simulink model "TVModel"  (R2022a)
settings: Solver=FixedStepDiscrete  StartTime=0.0  StopTime=10.0  FixedStep=0.02  MaxStep=0.01  RelTol=1e-3
undefined symbols (not defined in the file or in its folder): MB, TV, TV_OLD
libraries: simulink x22, simulink_extras x14, slpidlib x8, fuzblock x5, controlLib x4, dspstat3 x4, eeGeneralControl x3, cstblocks x3, eeSlidingModeController x1, sharedTrackingLibrary x1
(part 3 of 8)

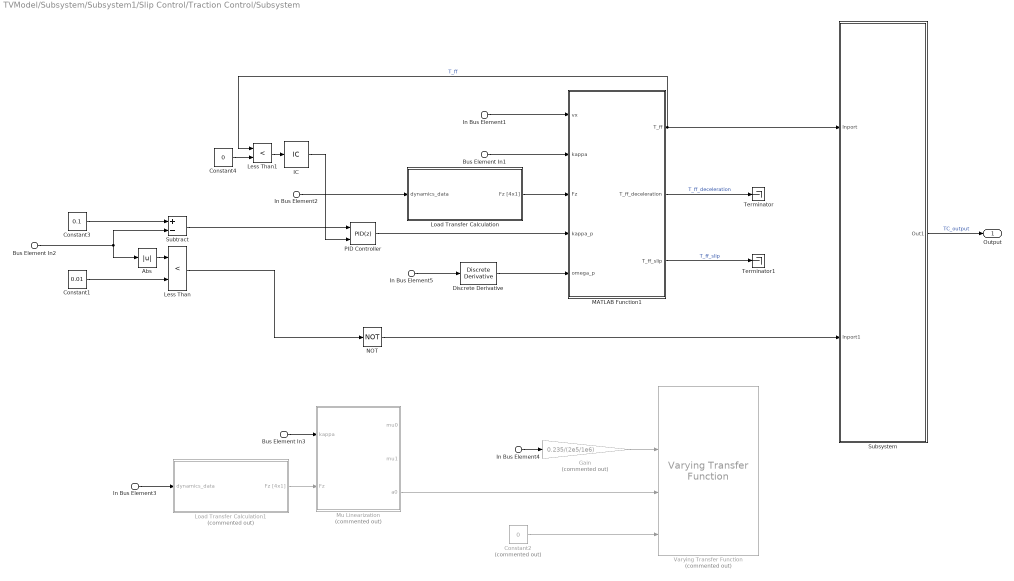
== system TVModel/Subsystem/Subsystem1/Slip Control/Traction Control/Subsystem ==
  In Bus Element2 : Inport  PortName=dynamics_data
  In Bus Element3 : Inport  PortName=dynamics_data
  In Bus Element1 : Inport  PortName=dynamics_data  Element=vx
  In Bus Element4 : Inport  PortName=dynamics_data  Element=vx
  In Bus Element5 : Inport  PortName=dynamics_data  Element=omega_wheels
  Bus Element In1 : Inport  Port=2  PortName=slip_ratio
  Bus Element In2 : Inport  Port=2  PortName=slip_ratio
  Bus Element In3 : Inport  Port=2  PortName=slip_ratio
  Abs : Abs  SaturateOnIntegerOverflow=off
  Constant1 : Constant  Value=0.01
  Constant2 : Constant  Commented=on  Value=0
  Constant3 : Constant  Value=0.1
  Constant4 : Constant  Value=0
  Discrete Derivative : simulink/Discrete/Discrete Derivative  gainval=1.0  ICPrevScaledInput=0.0  OutMin=[]  OutMax=[]  OutDataType=fixdt(1, 16)  OutScaling=2^-10  DoSatur=off
  Gain : Gain  Commented=on  Gain=0.235/(2e5/1e6)
  IC : InitialCondition
  Less Than : RelationalOperator  Operator=<  OutDataTypeStr=boolean  RndMeth=Simplest  InputSameDT=off
  Less Than1 : RelationalOperator  Operator=<  OutDataTypeStr=boolean  RndMeth=Simplest  InputSameDT=off
  Load Transfer Calculation : Subsystem
  Load Transfer Calculation1 : Subsystem  Commented=on
  MATLAB Function1 : MATLAB Function  TreatAsAtomicUnit=on
  Mu Linearization : MATLAB Function  Commented=on  TreatAsAtomicUnit=on
  NOT : Logic  Operator=NOT  IconShape=distinctive  AllPortsSameDT=off  OutDataTypeStr=boolean
  PID Controller : slpidlib/PID Controller  Controller=PID  Form=Parallel  TimeDomain=Discrete-time  UseExternalTs=off  SampleTime=-1  IntegratorMethod=Forward Euler  FilterMethod=Forward Euler  ControllerParametersSource=internal  P=1/(0.02*3)  I=100  UseKiTs=off  D=0  N=100  UseFilter=on  TunerSelectOption=Transfer Function Based (PID Tuner App)  InitialConditionSource=internal  InitialConditionForIntegrator=0  InitialConditionForFilter=0  DifferentiatorICPrevScaledInput=0  ExternalReset=level  TrackingMode=off  Kt=1  LimitOutput=on  SatLimitsSource=internal  UpperSaturationLimit=+20  LowerSaturationLimit=-20  LinearizeAsGain=on  AntiWindupMode=clamping  Kb=1  POutMin=[]  POutMax=[]  IOutMin=[]  IOutMax=[]  DOutMin=[]  DOutMax=[]  NOutMin=[]  NOutMax=[]  SumOutMin=[]  SumOutMax=[]  SaturationOutMin=[]  SaturationOutMax=[]  PParamMin=[]  PParamMax=[]  IParamMin=[]  IParamMax=[]  DParamMin=[]  DParamMax=[]  NParamMin=[]  NParamMax=[]  KbParamMin=[]  KbParamMax=[]  KtParamMin=[]  KtParamMax=[]  KbOutMin=[]  KbOutMax=[]  KtOutMin=[]  KtOutMax=[]  IntegratorOutMin=[]  IntegratorOutMax=[]  FilterOutMin=[]  FilterOutMax=[]  SumI1OutMin=[]  SumI1OutMax=[]  SumI2OutMin=[]  SumI2OutMax=[]  SumI3OutMin=[]  SumI3OutMax=[]  SumI4OutMin=[]  SumI4OutMax=[]  SumDOutMin=[]  SumDOutMax=[]  DifferentiatorOutMin=[]  DifferentiatorOutMax=[]  FilterDiffOutCoefMin=[]  FilterDiffOutCoefMax=[]  ReciprocalOutMin=[]  ReciprocalOutMax=[]  SumDenOutMin=[]  SumDenOutMax=[]  SumNumOutMin=[]  SumNumOutMax=[]  DivideOutMin=[]  DivideOutMax=[]  UdiffTsProdOutMin=[]  UdiffTsProdOutMax=[]  NTsProdOutMin=[]  NTsProdOutMax=[]  UintegralTsProdOutMin=[]  UintegralTsProdOutMax=[]  UngainTsProdOutMin=[]  UngainTsProdOutMax=[]  IntegratorContinuousStateAttributes=''  IntegratorStateMustResolveToSignalObject=off  IntegratorRTWStateStorageClass=Auto  FilterContinuousStateAttributes=''  FilterStateMustResolveToSignalObject=off  FilterRTWStateStorageClass=Auto  ParallelPVariant=InternalParameters  IdealPVariant=Disabled  IVariant=InternalParameters  DVariant=InternalParameters  IntegratorVariant=Discrete  SatVariant=Enabled  AWVariant=DiscClampingParallel  PCopyVariant=Disabled  TRVariant=Disabled  FdbkBlocksVariant=Forward  IdealPFdbkVariant=Disabled  SatFdbkVariant=Disabled  DerivativeFilterVariant=ForwardEulerFilter  NVariant=InternalParameters  NCopyVariant=Disabled  FilterICVariant=InternalICsFilter  IntegratorICVariant=InternalICs  ExternalResetVariant=ExternalReset  TRSumVariant=Passthrough  SumFdbkVariant=Disabled  SumVariant=Sum_PID  TsampFilterVariant=InternalTs  TsampNgainVariant=Passthrough  TsampIntegralVariant=Passthrough  ExternalSaturationOutDataTypeStr=Inherit: Same as second input  aMode=0
  Subsystem : Subsystem
  Subtract : Sum  Inputs=+-
  Terminator : Terminator
  Terminator1 : Terminator
  Varying Transfer Function : cstblocks/Linear Parameter Varying/Varying Transfer Function  Commented=on  N=1
  Output : Outport
  wires:
  Load Transfer Calculation/1(Fz [4x1]) -> MATLAB Function1/3(Fz)
  MATLAB Function1/1(T_ff) -> Less Than1/1, Subsystem/1(Inport)  "T_ff"
  Bus Element In1/1 -> MATLAB Function1/2(kappa)
  In Bus Element1/1 -> MATLAB Function1/1(vx)
  In Bus Element2/1 -> Load Transfer Calculation/1(dynamics_data)
  Bus Element In2/1 -> Subtract/2, Abs/1
  Constant3/1 -> Subtract/1
  Abs/1 -> Less Than/1
  Constant1/1 -> Less Than/2
  Subtract/1 -> PID Controller/1
  Bus Element In3/1 -> Mu Linearization/1(kappa)
  Load Transfer Calculation1/1(Fz [4x1]) -> Mu Linearization/2(Fz)
  In Bus Element3/1 -> Load Transfer Calculation1/1(dynamics_data)
  Constant2/1 -> Varying Transfer Function/4
  In Bus Element4/1 -> Gain/1
  Gain/1 -> Varying Transfer Function/2
  Mu Linearization/3(a0) -> Varying Transfer Function/3
  In Bus Element5/1 -> Discrete Derivative/1
  MATLAB Function1/2(T_ff_deceleration) -> Terminator/1  "T_ff_deceleration"
  MATLAB Function1/3(T_ff_slip) -> Terminator1/1  "T_ff_slip"
  Discrete Derivative/1 -> MATLAB Function1/5(omega_p)
  PID Controller/1 -> MATLAB Function1/4(kappa_p)
  NOT/1 -> Subsystem/2(Inport1)
  Subsystem/1(Out1) -> Output/1  "TC_output"
  Constant4/1 -> Less Than1/2
  Less Than1/1 -> IC/1
  Less Than/1 -> NOT/1
  IC/1 -> PID Controller/2

== system TVModel/Subsystem/Subsystem1/Slip Control/Traction Control/Subsystem1 ==
  In Bus Element2 : Inport  PortName=dynamics_data
  In Bus Element3 : Inport  PortName=dynamics_data
  In Bus Element1 : Inport  PortName=dynamics_data  Element=vx
  In Bus Element4 : Inport  PortName=dynamics_data  Element=vx
  In Bus Element5 : Inport  PortName=dynamics_data  Element=omega_wheels
  Bus Element In1 : Inport  Port=2  PortName=slip_ratio
  Bus Element In2 : Inport  Port=2  PortName=slip_ratio
  Bus Element In3 : Inport  Port=2  PortName=slip_ratio
  Abs : Abs  SaturateOnIntegerOverflow=off
  Constant1 : Constant  Value=0.01
  Constant2 : Constant  Commented=on  Value=0
  Constant3 : Constant  Value=-0.1
  Discrete Derivative : simulink/Discrete/Discrete Derivative  gainval=1.0  ICPrevScaledInput=0.0  OutMin=[]  OutMax=[]  OutDataType=fixdt(1, 16)  OutScaling=2^-10  DoSatur=off
  Gain : Gain  Commented=on  Gain=0.235/(2e5/1e6)
  Less Than : RelationalOperator  Operator=<  OutDataTypeStr=boolean  RndMeth=Simplest  InputSameDT=off
  Load Transfer Calculation : Subsystem
  Load Transfer Calculation1 : Subsystem  Commented=on
  MATLAB Function1 : MATLAB Function  TreatAsAtomicUnit=on
  Mu Linearization : MATLAB Function  Commented=on  TreatAsAtomicUnit=on
  NOT : Logic  Operator=NOT  IconShape=distinctive  AllPortsSameDT=off  OutDataTypeStr=boolean
  PID Controller : slpidlib/PID Controller  Controller=PID  Form=Parallel  TimeDomain=Discrete-time  UseExternalTs=off  SampleTime=-1  IntegratorMethod=Forward Euler  FilterMethod=Forward Euler  ControllerParametersSource=internal  P=1/(0.02*3)  I=100  UseKiTs=off  D=0  N=100  UseFilter=on  TunerSelectOption=Transfer Function Based (PID Tuner App)  InitialConditionSource=internal  InitialConditionForIntegrator=0  InitialConditionForFilter=0  DifferentiatorICPrevScaledInput=0  ExternalReset=level  TrackingMode=off  Kt=1  LimitOutput=on  SatLimitsSource=internal  UpperSaturationLimit=-5  LowerSaturationLimit=-20  LinearizeAsGain=on  AntiWindupMode=clamping  Kb=1  POutMin=[]  POutMax=[]  IOutMin=[]  IOutMax=[]  DOutMin=[]  DOutMax=[]  NOutMin=[]  NOutMax=[]  SumOutMin=[]  SumOutMax=[]  SaturationOutMin=[]  SaturationOutMax=[]  PParamMin=[]  PParamMax=[]  IParamMin=[]  IParamMax=[]  DParamMin=[]  DParamMax=[]  NParamMin=[]  NParamMax=[]  KbParamMin=[]  KbParamMax=[]  KtParamMin=[]  KtParamMax=[]  KbOutMin=[]  KbOutMax=[]  KtOutMin=[]  KtOutMax=[]  IntegratorOutMin=[]  IntegratorOutMax=[]  FilterOutMin=[]  FilterOutMax=[]  SumI1OutMin=[]  SumI1OutMax=[]  SumI2OutMin=[]  SumI2OutMax=[]  SumI3OutMin=[]  SumI3OutMax=[]  SumI4OutMin=[]  SumI4OutMax=[]  SumDOutMin=[]  SumDOutMax=[]  DifferentiatorOutMin=[]  DifferentiatorOutMax=[]  FilterDiffOutCoefMin=[]  FilterDiffOutCoefMax=[]  ReciprocalOutMin=[]  ReciprocalOutMax=[]  SumDenOutMin=[]  SumDenOutMax=[]  SumNumOutMin=[]  SumNumOutMax=[]  DivideOutMin=[]  DivideOutMax=[]  UdiffTsProdOutMin=[]  UdiffTsProdOutMax=[]  NTsProdOutMin=[]  NTsProdOutMax=[]  UintegralTsProdOutMin=[]  UintegralTsProdOutMax=[]  UngainTsProdOutMin=[]  UngainTsProdOutMax=[]  IntegratorContinuousStateAttributes=''  IntegratorStateMustResolveToSignalObject=off  IntegratorRTWStateStorageClass=Auto  FilterContinuousStateAttributes=''  FilterStateMustResolveToSignalObject=off  FilterRTWStateStorageClass=Auto  ParallelPVariant=InternalParameters  IdealPVariant=Disabled  IVariant=InternalParameters  DVariant=InternalParameters  IntegratorVariant=Discrete  SatVariant=Enabled  AWVariant=DiscClampingParallel  PCopyVariant=Disabled  TRVariant=Disabled  FdbkBlocksVariant=Forward  IdealPFdbkVariant=Disabled  SatFdbkVariant=Disabled  DerivativeFilterVariant=ForwardEulerFilter  NVariant=InternalParameters  NCopyVariant=Disabled  FilterICVariant=InternalICsFilter  IntegratorICVariant=InternalICs  ExternalResetVariant=ExternalReset  TRSumVariant=Passthrough  SumFdbkVariant=Disabled  SumVariant=Sum_PID  TsampFilterVariant=InternalTs  TsampNgainVariant=Passthrough  TsampIntegralVariant=Passthrough  ExternalSaturationOutDataTypeStr=Inherit: Same as second input  aMode=0
  Subsystem : Subsystem
  Subtract : Sum  Inputs=+-
  Terminator : Terminator
  Terminator1 : Terminator
  Varying Transfer Function : cstblocks/Linear Parameter Varying/Varying Transfer Function  Commented=on  N=1
  Output : Outport
  wires:
  Load Transfer Calculation/1(Fz [4x1]) -> MATLAB Function1/3(Fz)
  MATLAB Function1/1(T_ff) -> Subsystem/1(Inport)  "T_ff"
  Bus Element In1/1 -> MATLAB Function1/2(kappa)
  In Bus Element1/1 -> MATLAB Function1/1(vx)
  In Bus Element2/1 -> Load Transfer Calculation/1(dynamics_data)
  Bus Element In2/1 -> Subtract/2, Abs/1
  Constant3/1 -> Subtract/1
  Less Than/1 -> PID Controller/2, NOT/1
  Abs/1 -> Less Than/1
  Constant1/1 -> Less Than/2
  Subtract/1 -> PID Controller/1
  Bus Element In3/1 -> Mu Linearization/1(kappa)
  Load Transfer Calculation1/1(Fz [4x1]) -> Mu Linearization/2(Fz)
  In Bus Element3/1 -> Load Transfer Calculation1/1(dynamics_data)
  Constant2/1 -> Varying Transfer Function/4
  In Bus Element4/1 -> Gain/1
  Gain/1 -> Varying Transfer Function/2
  Mu Linearization/3(a0) -> Varying Transfer Function/3
  In Bus Element5/1 -> Discrete Derivative/1
  MATLAB Function1/2(T_ff_deceleration) -> Terminator/1  "T_ff_deceleration"
  MATLAB Function1/3(T_ff_slip) -> Terminator1/1  "T_ff_slip"
  Discrete Derivative/1 -> MATLAB Function1/5(omega_p)
  PID Controller/1 -> MATLAB Function1/4(kappa_p)
  NOT/1 -> Subsystem/2(Inport1)
  Subsystem/1(Out1) -> Output/1  "TC_output"

== system TVModel/Subsystem/Subsystem1/Torque Distribution/MPC/     Output Vector Reference ==
  YRD : Inport
  Bus Creator : BusCreator  Inputs=11
  T_FL_ref : Constant  Value=0
  T_FR_ref : Constant  Value=0
  T_RL_ref : Constant  Value=0
  T_RR_ref : Constant  Value=0
  VX_ref : Constant  Value=0
  VY_ref : Constant  Value=0
  Vector Concatenate : Concatenate
  dT_FL_ref : Constant  Value=0
  dT_FR_ref : Constant  Value=0
  dT_RL_ref : Constant  Value=0
  dT_RR_ref : Constant  Value=0
  y_ref_e : Outport
  Out Bus Element2 : Outport  Port=2  PortName=TV_Info  Element=y_ref
  wires:
  dT_RR_ref/1 -> Bus Creator/11  "dt_rr_ref"
  dT_RL_ref/1 -> Bus Creator/10  "dt_rl_ref"
  dT_FR_ref/1 -> Bus Creator/9  "dt_fr_ref"
  dT_FL_ref/1 -> Bus Creator/8  "dt_fl_ref"
  VX_ref/1 -> Bus Creator/1  "vx_ref"
  VY_ref/1 -> Bus Creator/2  "vy_ref"
  T_FL_ref/1 -> Bus Creator/4  "t_fl_ref"
  T_FR_ref/1 -> Bus Creator/5  "t_fr_ref"
  T_RL_ref/1 -> Bus Creator/6  "t_rl_ref"
  T_RR_ref/1 -> Bus Creator/7  "t_rr_ref"
  Bus Creator/1 -> Vector Concatenate/2, Vector Concatenate/1
  YRD/1 -> Bus Creator/3  "r_ref"
  Vector Concatenate/1 -> y_ref_e/1

== system TVModel/Subsystem/Subsystem1/Torque Distribution/MPC/ PRE LUDO ==
  Brake & ESP : Subsystem
  Cross Check1 : MATLAB Function  TreatAsAtomicUnit=on
  Faul Detection : Subsystem
  Hydraulic brakes : Subsystem
  Mz = 0 Bound logic : Subsystem
  Power Calculation Post : Subsystem  Commented=on
  Power Calculation Pre : Subsystem  Commented=on
  Steer_activation : Subsystem  Commented=on

== system TVModel/Subsystem/Subsystem1/Torque Distribution/MPC/ Parameter Bus  ==
  In Bus Element1 : Inport  PortName=slip_ratio  Element=fl
  In Bus Element2 : Inport  PortName=slip_ratio  Element=fr
  In Bus Element3 : Inport  PortName=slip_ratio  Element=rl
  In Bus Element4 : Inport  PortName=slip_ratio  Element=rr
  In Bus Element5 : Inport  Port=2  PortName=dynamics_data  Element=ax
  In Bus Element6 : Inport  Port=2  PortName=dynamics_data  Element=ay
  In Bus Element12 : Inport  Port=2  PortName=dynamics_data  Element=brake_torque
  In Bus Element11 : Inport  Port=3  PortName=front_wheel_angles  Element=single_axis
  Bus p : Subsystem
  Demux : Demux
  Inertia Scaling : Constant  Value=TV.SIGNALS.SETTINGS.IzScale
  LMUy : Constant  Value=TV.SIGNALS.SETTINGS.LMU
  Mux : Mux  Inputs=TV.MPC.np
  Signal Specification{4..7} (4 alike) : SignalSpecification  Dimensions=1
  p : Outport
  Out Bus Element6 : Outport  Port=2  PortName=TV_Info  Element=p
  wires:
  Inertia Scaling/1 -> Mux/13  "iz_scale"
  In Bus Element11/1 -> Mux/1  "wheel_angle_single_axis"
  LMUy/1 -> Mux/12  "lmu"
  Bus p/1(TV_Info) -> Out Bus Element6/1, p/1
  Demux/1 -> Signal Specification4/1
  Demux/2 -> Signal Specification5/1
  Demux/3 -> Signal Specification6/1
  Demux/4 -> Signal Specification7/1
  Signal Specification4/1 -> Mux/6  "brake_torque_fl"
  Signal Specification5/1 -> Mux/7  "brake_torque_fr"
  Signal Specification6/1 -> Mux/8  "brake_torque_rl"
  Signal Specification7/1 -> Mux/9  "brake_torque_rr"
  Mux/1 -> Bus p/1(In)
  In Bus Element1/1 -> Mux/2  "slip_ratio_fl"
  In Bus Element4/1 -> Mux/5  "slip_ratio_rr"
  In Bus Element3/1 -> Mux/4  "slip_ratio_rl"
  In Bus Element2/1 -> Mux/3  "slip_ratio_fr"
  In Bus Element6/1 -> Mux/10  "ay"
  In Bus Element5/1 -> Mux/11  "ax"
  In Bus Element12/1 -> Demux/1

== system TVModel/Subsystem/Subsystem1/Torque Distribution/MPC/ States ==
  motor_torque : Inport
  In Bus Element : Inport  Port=2  PortName=dynamics_data  Element=vx
  In Bus Element1 : Inport  Port=2  PortName=dynamics_data  Element=vy
  In Bus Element2 : Inport  Port=2  PortName=dynamics_data  Element=yaw_rate
  Bus Creator1 : BusCreator  Inputs=7
  Demux : Demux
  Saturation : Saturate  UpperLimit=inf  LowerLimit=2
  Saturation1 : Saturate  UpperLimit=5  LowerLimit=-5
  Saturation2 : Saturate  UpperLimit=4  LowerLimit=-4
  x : Outport
  Out Bus Element6 : Outport  Port=2  PortName=TV_Info  Element=x
  wires:
  In Bus Element2/1 -> Saturation2/1
  Saturation/1 -> Bus Creator1/1  "vx"
  In Bus Element1/1 -> Saturation1/1
  In Bus Element/1 -> Saturation/1
  Bus Creator1/1 -> Out Bus Element6/1, x/1
  Saturation1/1 -> Bus Creator1/2  "vy"
  Saturation2/1 -> Bus Creator1/3  "yaw_rate"
  motor_torque/1 -> Demux/1
  Demux/4 -> Bus Creator1/7  "t_rr"
  Demux/3 -> Bus Creator1/6  "t_rl"
  Demux/2 -> Bus Creator1/5  "t_fr"
  Demux/1 -> Bus Creator1/4  "t_fl"

== system TVModel/Subsystem/Subsystem1/Torque Distribution/MPC/Control Constraints ==
  Constant : Constant  Value=10000*ones(4,1)
  Unary Minus : UnaryMinus
  lbu : Outport
  ubu : Outport  Port=2
  Out Bus Element19 : Outport  Port=3  PortName=TV_Info  Element=lbu
  Out Bus Element1 : Outport  Port=3  PortName=TV_Info  Element=ubu
  wires:
  Unary Minus/1 -> Out Bus Element19/1, lbu/1
  Constant/1 -> Out Bus Element1/1, ubu/1, Unary Minus/1

== system TVModel/Subsystem/Subsystem1/Torque Distribution/MPC/Faults Detection ==
  OCP Status : Inport
  In Bus throttle : Inport  Port=2  PortName=driver_inputs
  In Bus throttle1 : Inport  Port=2  PortName=driver_inputs
  In Bus Element1 : Inport  Port=2  PortName=driver_inputs  Element=throttle
  In Bus Element4 : Inport  Port=2  PortName=driver_inputs  Element=brake
  In Bus Element2 : Inport  Port=3  PortName=dynamics_data
  In Bus Element3 : Inport  Port=3  PortName=dynamics_data
  In Bus Element7 : Inport  Port=3  PortName=dynamics_data
  In Bus Element6 : Inport  Port=4  PortName=brake_signal
  In Bus Element8 : Inport  Port=4  PortName=brake_signal
  In Bus Element9 : Inport  Port=5  PortName=hv
  In Bus torque_map3 : Inport  Port=6  PortName=car_settings
  X1 : Inport  Port=7
  Constant : Constant
  Data Store General_Params1 : DataStoreRead  DataStoreName=General_Params  DataStoreElements=General_Params.BrakeThresh  IndexOptions=Index vector (dialog)  Indices=1  OutputSizes=1
  Divide : Product  Inputs=**
  If : If  IfExpression=u1 == 1  ElseIfExpressions=u1 == 2
  Less Than3 : RelationalOperator  Operator=>  OutDataTypeStr=boolean  RndMeth=Simplest  InputSameDT=off
  MPC : Subsystem  TreatAsAtomicUnit=on
  Merge : Merge  Inputs=3
  Overlap Chart : Stateflow chart  TreatAsAtomicUnit=on
  Selector : Selector  InputPortWidth=7  IndexOptions=Index vector (dialog)  Indices=[4:7]  OutputSizes=1
  Simple torque : Subsystem  TreatAsAtomicUnit=on
  Subsystem : Subsystem
  Vectorino : Subsystem  TreatAsAtomicUnit=on
  Torque : Outport
  Out Bus Element8 : Outport  Port=2  PortName=TV_Info  Element=torque_flag
  wires:
  Constant/1 -> Divide/2
  In Bus Element1/1 -> Overlap Chart/1(throttle)  "throttle_pre"
  In Bus Element4/1 -> Less Than3/1
  Divide/1 -> Torque/1
  Overlap Chart/1(torque_flag) -> Out Bus Element8/1
  Less Than3/1 -> Overlap Chart/2(brake)
  Data Store General_Params1/1 -> Less Than3/2
  In Bus throttle1/1 -> Vectorino/2(driver_inputs)
  In Bus Element8/1 -> Vectorino/3(brake_signal)
  Vectorino/1(Output) -> Merge/2
  In Bus Element3/1 -> Vectorino/1(dynamics_data)
  Selector/1 -> MPC/1(In1)  "Torque"
  If/2 -> Vectorino/Action
  Subsystem/1(TV Mode Selection) -> If/1  "Mode_Selector"
  X1/1 -> Selector/1
  If/3 -> Simple torque/Action
  If/1 -> MPC/Action
  OCP Status/1 -> Subsystem/1(OCP Status)
  Simple torque/1(Out1) -> Merge/3
  MPC/1(Out1) -> Merge/1
  Merge/1 -> Divide/1
  In Bus throttle/1 -> Simple torque/1(driver_inputs)
  In Bus Element2/1 -> Simple torque/2(dynamics_data)
  In Bus Element9/1 -> Simple torque/4(hv)
  In Bus Element6/1 -> Simple torque/3(brake_signal)
  In Bus torque_map3/1 -> Simple torque/5(car_settings)
  In Bus Element7/1 -> Subsystem/2(dynamics_data)

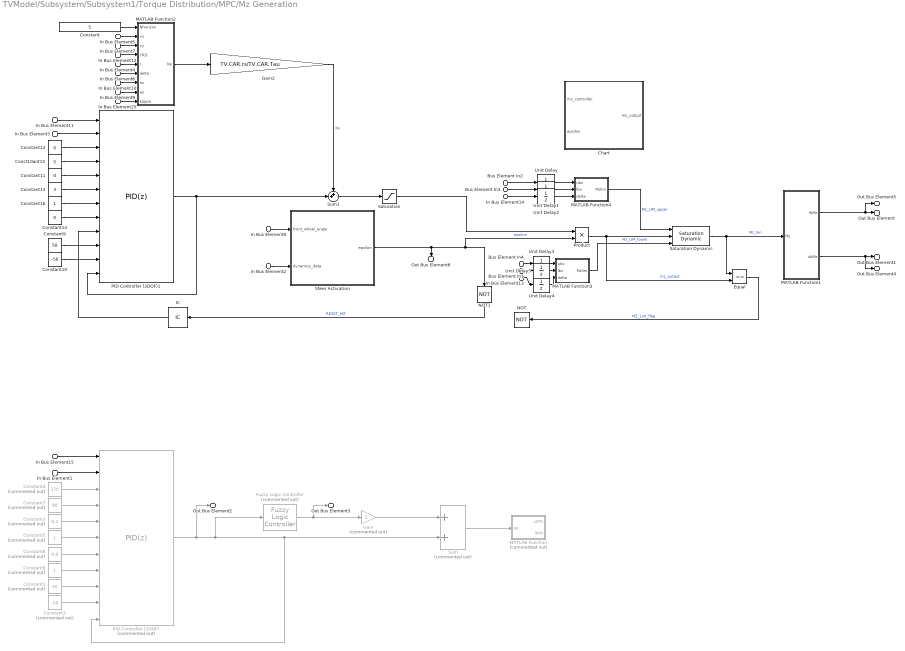
== system TVModel/Subsystem/Subsystem1/Torque Distribution/MPC/Mz Generation ==
  In Bus Element2 : Inport  PortName=dynamics_data
  In Bus Element1 : Inport  PortName=dynamics_data  Element=yaw_rate
  In Bus Element3 : Inport  PortName=dynamics_data  Element=yaw_rate
  In Bus Element4 : Inport  PortName=dynamics_data  Element=yaw_rate
  In Bus Element5 : Inport  PortName=dynamics_data  Element=vx
  In Bus Element7 : Inport  PortName=dynamics_data  Element=vy
  In Bus Element9 : Inport  PortName=dynamics_data  Element=ay
  In Bus Element10 : Inport  PortName=dynamics_data  Element=ax
  In Bus Element8 : Inport  Port=2  PortName=front_wheel_angles  Element=single_axis
  In Bus Element6 : Inport  Port=2  PortName=front_wheel_angles  Element=single_axis
  In Bus Element14 : Inport  Port=2  PortName=front_wheel_angles  Element=different_axis
  In Bus Element13 : Inport  Port=2  PortName=front_wheel_angles  Element=different_axis
  In Bus Element25 : Inport  Port=3  PortName=slip_ratio
  In Bus Element15 : Inport  Port=4  PortName=yaw_rate_desired
  In Bus Element11 : Inport  Port=4  PortName=yaw_rate_desired
  In Bus Element12 : Inport  Port=4  PortName=yaw_rate_desired
  Bus Element In3 : Inport  Port=5  PortName=Torque_Bounds  Element=lbx
  Bus Element In1 : Inport  Port=5  PortName=Torque_Bounds  Element=lbx
  Bus Element In2 : Inport  Port=5  PortName=Torque_Bounds  Element=ubx
  Bus Element In4 : Inport  Port=5  PortName=Torque_Bounds  Element=ubx
  Chart : Stateflow chart  TreatAsAtomicUnit=on
  Const10ant15 : Constant  Value=5
  Constant : Constant  Value=5
  Constant1 : Constant  Commented=on  Value=50
  Constant10 : Constant  Value=-50
  Constant11 : Constant  Value=0
  Constant12 : Constant  Value=0
  Constant13 : Constant  Value=3
  Constant14 : Constant  Value=0
  Constant16 : Constant
  Constant2 : Constant  Commented=on  Value=-50
  Constant3 : Constant  Commented=on  Value=0.3
  Constant4 : Constant  Commented=on  Value=170
  Constant5 : Constant  Commented=on
  Constant6 : Constant  Commented=on
  Constant7 : Constant  Commented=on  Value=90
  Constant8 : Constant  Commented=on  Value=0.9
  Constant9 : Constant  Value=50
  Equal : RelationalOperator  Operator===  OutDataTypeStr=boolean  RndMeth=Simplest  InputSameDT=off
  Fuzzy Logic Controller : fuzblock/Fuzzy Logic  Controller  Commented=on  FIS='Fuzzy_Reference.fis'  OutputSampleNumber=101  DataType=double  FuzzifiedInputs=off  RuleFiringStrengths=off  RuleOutputs=off  AggregatedOutputs=off  SimulateUsing=Interpreted execution  OutOfRangeInputValueMessage=warning  NoRuleFiredMessage=warning  EmptyOutputFuzzySetMessage=warning
  Gain : Gain  Commented=on  Gain=2
  Gain2 : Gain  Gain=TV.CAR.rs/TV.CAR.Tau
  IC : InitialCondition
  MATLAB Function : MATLAB Function  Commented=on  TreatAsAtomicUnit=on
  MATLAB Function1 : MATLAB Function  TreatAsAtomicUnit=on
  MATLAB Function2 : MATLAB Function  TreatAsAtomicUnit=on
  MATLAB Function3 : MATLAB Function  TreatAsAtomicUnit=on
  MATLAB Function4 : MATLAB Function  TreatAsAtomicUnit=on
  NOT : Logic  Operator=NOT  IconShape=distinctive  AllPortsSameDT=off  OutDataTypeStr=boolean
  NOT1 : Logic  Operator=NOT  IconShape=distinctive  AllPortsSameDT=off  OutDataTypeStr=boolean
  PID Controller (2DOF) : slpidlib/PID Controller (2DOF)  Commented=on  Controller=PID  Form=Parallel  TimeDomain=Discrete-time  UseExternalTs=off  SampleTime=0.02  IntegratorMethod=Forward Euler  FilterMethod=Forward Euler  ControllerParametersSource=external  P=1  I=1  UseKiTs=off  D=0  N=100  UseFilter=on  b=1  c=1  TunerSelectOption=Transfer Function Based (PID Tuner App)  InitialConditionSource=internal  InitialConditionForIntegrator=0  InitialConditionForFilter=0  DifferentiatorICPrevScaledInput=0  ExternalReset=none  TrackingMode=on  Kt=100  LimitOutput=on  SatLimitsSource=external  UpperSaturationLimit=inf  LowerSaturationLimit=-inf  LinearizeAsGain=on  AntiWindupMode=clamping  Kb=100  POutMin=[]  POutMax=[]  IOutMin=[]  IOutMax=[]  DOutMin=[]  DOutMax=[]  NOutMin=[]  NOutMax=[]  bOutMin=[]  bOutMax=[]  cOutMin=[]  cOutMax=[]  SumOutMin=[]  SumOutMax=[]  SaturationOutMin=[]  SaturationOutMax=[]  PParamMin=[]  PParamMax=[]  IParamMin=[]  IParamMax=[]  DParamMin=[]  DParamMax=[]  NParamMin=[]  NParamMax=[]  bParamMin=[]  bParamMax=[]  cParamMin=[]  cParamMax=[]  KbParamMin=[]  KbParamMax=[]  KtParamMin=[]  KtParamMax=[]  KbOutMin=[]  KbOutMax=[]  KtOutMin=[]  KtOutMax=[]  IntegratorOutMin=[]  IntegratorOutMax=[]  FilterOutMin=[]  FilterOutMax=[]  SumI1OutMin=[]  SumI1OutMax=[]  SumI2OutMin=[]  SumI2OutMax=[]  SumI3OutMin=[]  SumI3OutMax=[]  SumI4OutMin=[]  SumI4OutMax=[]  SumDOutMin=[]  SumDOutMax=[]  Sum1OutMin=[]  Sum1OutMax=[]  Sum2OutMin=[]  Sum2OutMax=[]  Sum3OutMin=[]  Sum3OutMax=[]  DifferentiatorOutMin=[]  DifferentiatorOutMax=[]  FilterDiffOutCoefMin=[]  FilterDiffOutCoefMax=[]  ReciprocalOutMin=[]  ReciprocalOutMax=[]  SumDenOutMin=[]  SumDenOutMax=[]  SumNumOutMin=[]  SumNumOutMax=[]  DivideOutMin=[]  DivideOutMax=[]  UdiffTsProdOutMin=[]  UdiffTsProdOutMax=[]  NTsProdOutMin=[]  NTsProdOutMax=[]  UintegralTsProdOutMin=[]  UintegralTsProdOutMax=[]  UngainTsProdOutMin=[]  UngainTsProdOutMax=[]  IntegratorContinuousStateAttributes=''  IntegratorStateMustResolveToSignalObject=off  IntegratorRTWStateStorageClass=Auto  FilterContinuousStateAttributes=''  FilterStateMustResolveToSignalObject=off  FilterRTWStateStorageClass=Auto  ParallelPVariant=ExternalParameters  IdealPVariant=Disabled  IVariant=ExternalParameters  DVariant=ExternalParameters  bVariant=ExternalParameters  cVariant=ExternalParameters  IntegratorVariant=Discrete  SatVariant=External  AWVariant=DiscClampingParallel  PCopyVariant=Disabled  TRVariant=Enabled  FdbkBlocksVariant=Forward  IdealPFdbkVariant=Disabled  SatFdbkVariant=Disabled  DerivativeFilterVariant=ForwardEulerFilter  NVariant=ExternalParameters  NCopyVariant=Disabled  FilterICVariant=InternalICsFilter  IntegratorICVariant=InternalICs  ExternalResetVariant=Disabled  TRSumVariant=TrackingMode  SumFdbkVariant=Disabled  SumVariant=Sum_PID  TsampFilterVariant=InternalTs  TsampNgainVariant=Passthrough  TsampIntegralVariant=Passthrough  ExternalSaturationOutDataTypeStr=Inherit: Same as second input
      settings: SourceProductBaseCode=SL
  PID Controller (2DOF)1 : slpidlib/PID Controller (2DOF)  Controller=PID  Form=Parallel  TimeDomain=Discrete-time  UseExternalTs=off  SampleTime=0.02  IntegratorMethod=Forward Euler  FilterMethod=Forward Euler  ControllerParametersSource=external  P=1  I=1  UseKiTs=off  D=0  N=100  UseFilter=on  b=1  c=1  TunerSelectOption=Transfer Function Based (PID Tuner App)  InitialConditionSource=internal  InitialConditionForIntegrator=0  InitialConditionForFilter=0  DifferentiatorICPrevScaledInput=0  ExternalReset=level  TrackingMode=on  Kt=100  LimitOutput=on  SatLimitsSource=external  UpperSaturationLimit=inf  LowerSaturationLimit=-inf  LinearizeAsGain=on  AntiWindupMode=clamping  Kb=100  POutMin=[]  POutMax=[]  IOutMin=[]  IOutMax=[]  DOutMin=[]  DOutMax=[]  NOutMin=[]  NOutMax=[]  bOutMin=[]  bOutMax=[]  cOutMin=[]  cOutMax=[]  SumOutMin=[]  SumOutMax=[]  SaturationOutMin=[]  SaturationOutMax=[]  PParamMin=[]  PParamMax=[]  IParamMin=[]  IParamMax=[]  DParamMin=[]  DParamMax=[]  NParamMin=[]  NParamMax=[]  bParamMin=[]  bParamMax=[]  cParamMin=[]  cParamMax=[]  KbParamMin=[]  KbParamMax=[]  KtParamMin=[]  KtParamMax=[]  KbOutMin=[]  KbOutMax=[]  KtOutMin=[]  KtOutMax=[]  IntegratorOutMin=[]  IntegratorOutMax=[]  FilterOutMin=[]  FilterOutMax=[]  SumI1OutMin=[]  SumI1OutMax=[]  SumI2OutMin=[]  SumI2OutMax=[]  SumI3OutMin=[]  SumI3OutMax=[]  SumI4OutMin=[]  SumI4OutMax=[]  SumDOutMin=[]  SumDOutMax=[]  Sum1OutMin=[]  Sum1OutMax=[]  Sum2OutMin=[]  Sum2OutMax=[]  Sum3OutMin=[]  Sum3OutMax=[]  DifferentiatorOutMin=[]  DifferentiatorOutMax=[]  FilterDiffOutCoefMin=[]  FilterDiffOutCoefMax=[]  ReciprocalOutMin=[]  ReciprocalOutMax=[]  SumDenOutMin=[]  SumDenOutMax=[]  SumNumOutMin=[]  SumNumOutMax=[]  DivideOutMin=[]  DivideOutMax=[]  UdiffTsProdOutMin=[]  UdiffTsProdOutMax=[]  NTsProdOutMin=[]  NTsProdOutMax=[]  UintegralTsProdOutMin=[]  UintegralTsProdOutMax=[]  UngainTsProdOutMin=[]  UngainTsProdOutMax=[]  IntegratorContinuousStateAttributes=''  IntegratorStateMustResolveToSignalObject=off  IntegratorRTWStateStorageClass=Auto  FilterContinuousStateAttributes=''  FilterStateMustResolveToSignalObject=off  FilterRTWStateStorageClass=Auto  ParallelPVariant=ExternalParameters  IdealPVariant=Disabled  IVariant=ExternalParameters  DVariant=ExternalParameters  bVariant=ExternalParameters  cVariant=ExternalParameters  IntegratorVariant=Discrete  SatVariant=External  AWVariant=DiscClampingParallel  PCopyVariant=Disabled  TRVariant=Enabled  FdbkBlocksVariant=Forward  IdealPFdbkVariant=Disabled  SatFdbkVariant=Disabled  DerivativeFilterVariant=ForwardEulerFilter  NVariant=ExternalParameters  NCopyVariant=Disabled  FilterICVariant=InternalICsFilter  IntegratorICVariant=InternalICs  ExternalResetVariant=ExternalReset  TRSumVariant=TrackingMode  SumFdbkVariant=Disabled  SumVariant=Sum_PID  TsampFilterVariant=InternalTs  TsampNgainVariant=Passthrough  TsampIntegralVariant=Passthrough  ExternalSaturationOutDataTypeStr=Inherit: Same as second input
      settings: SourceProductBaseCode=SL
  Product : Product
  Saturation : Saturate  UpperLimit=15  LowerLimit=-15
  Saturation Dynamic : simulink/Discontinuities/Saturation Dynamic  OutMin=[]  OutMax=[]  OutDataTypeStr=Inherit: Same as second input  OutDataType=fixdt(1, 16)  OutScaling=2^-10  DoSatur=off
  Steer Activation : Subsystem
  Sum : Sum  Commented=on
  Sum1 : Sum  Inputs=++|
  Unit Delay{,1..5} (6 alike) : UnitDelay  SampleTime=-1  HasFrameUpgradeWarning=on
  Out Bus Element : Outport  PortName=mz  Element=lb
  Out Bus Element1 : Outport  PortName=mz  Element=ub
  Out Bus Element3 : Outport  Port=2  PortName=TV_Info  Element=fuzzy_out
  Out Bus Element2 : Outport  Port=2  PortName=TV_Info  Element=pid_out
  Out Bus Element4 : Outport  Port=2  PortName=TV_Info  Element=mz_ub
  Out Bus Element5 : Outport  Port=2  PortName=TV_Info  Element=mz_lb
  Out Bus Element6 : Outport  Port=3  PortName=epsilon
  wires:
  Bus Element In2/1 -> Unit Delay/1
  In Bus Element14/1 -> Unit Delay2/1
  Sum1/1 -> Saturation/1
  Product/1 -> Equal/2, Saturation Dynamic/2  "mz_output"
  Saturation Dynamic/1 -> Equal/1, MATLAB Function1/1(Mz)  "Mz_lim"
  Constant/1 -> MATLAB Function2/1(Nhorizon)
  Gain/1 -> Sum/1
  Fuzzy Logic Controller/1 -> Out Bus Element3/1, Gain/1
  Constant4/1 -> PID Controller (2DOF)/3
  Constant7/1 -> PID Controller (2DOF)/4
  PID Controller (2DOF)/1 -> Out Bus Element2/1, Sum/2, PID Controller (2DOF)/11, Fuzzy Logic Controller/1
  Constant1/1 -> PID Controller (2DOF)/9
  In Bus Element15/1 -> PID Controller (2DOF)/1
  In Bus Element1/1 -> PID Controller (2DOF)/2
  Constant2/1 -> PID Controller (2DOF)/10
  Constant8/1 -> PID Controller (2DOF)/7
  Sum/1 -> MATLAB Function/1(Mz)
  Constant3/1 -> PID Controller (2DOF)/5
  Constant5/1 -> PID Controller (2DOF)/6
  Constant6/1 -> PID Controller (2DOF)/8
  In Bus Element2/1 -> Steer Activation/2(dynamics_data)
  In Bus Element25/1 -> MATLAB Function2/9(kappa)
  Constant16/1 -> PID Controller (2DOF)1/7
  Constant14/1 -> PID Controller (2DOF)1/8
  In Bus Element6/1 -> MATLAB Function2/6(delta)
  Constant13/1 -> PID Controller (2DOF)1/6
  Const10ant15/1 -> PID Controller (2DOF)1/4
  In Bus Element5/1 -> MATLAB Function2/2(vx)
  Constant10/1 -> PID Controller (2DOF)1/11
  Steer Activation/1(epsilon) -> Out Bus Element6/1, NOT1/1, Product/2  "epsilon"
  Constant12/1 -> PID Controller (2DOF)1/3
  In Bus Element8/1 -> Steer Activation/1(front_wheel_angle)
  Constant9/1 -> PID Controller (2DOF)1/10
  MATLAB Function1/1(lbMz) -> Out Bus Element5/1, Out Bus Element/1
  In Bus Element4/1 -> MATLAB Function2/5(r)
  In Bus Element10/1 -> MATLAB Function2/7(ax)
  In Bus Element9/1 -> MATLAB Function2/8(ay)
  MATLAB Function2/1(Nx) -> Gain2/1
  MATLAB Function1/2(ubMz) -> Out Bus Element4/1, Out Bus Element1/1
  Gain2/1 -> Sum1/1  "Nx"
  In Bus Element3/1 -> PID Controller (2DOF)1/2
  Constant11/1 -> PID Controller (2DOF)1/5
  In Bus Element7/1 -> MATLAB Function2/3(vy)
  In Bus Element11/1 -> PID Controller (2DOF)1/1
  In Bus Element12/1 -> MATLAB Function2/4(YRD)
  PID Controller (2DOF)1/1 -> PID Controller (2DOF)1/12, Sum1/2
  Equal/1 -> NOT/1  "MZ_Lim_flag"
  Bus Element In3/1 -> Unit Delay1/1
  NOT1/1 -> IC/1  "RESET_MZ"
  MATLAB Function4/1(Mzlim) -> Saturation Dynamic/1  "Mz_LIM_upper"
  MATLAB Function3/1(Mzlim) -> Saturation Dynamic/3  "Mz_LIM_lower"
  Unit Delay/1 -> MATLAB Function4/1(ubx)
  Unit Delay1/1 -> MATLAB Function4/2(lbx)
  Unit Delay2/1 -> MATLAB Function4/3(delta)
  Unit Delay3/1 -> MATLAB Function3/1(ubx)
  Bus Element In4/1 -> Unit Delay3/1
  In Bus Element13/1 -> Unit Delay4/1
  Unit Delay4/1 -> MATLAB Function3/3(delta)
  Bus Element In1/1 -> Unit Delay5/1
  Unit Delay5/1 -> MATLAB Function3/2(lbx)
  Saturation/1 -> Product/1
  IC/1 -> PID Controller (2DOF)1/9

== system TVModel/Subsystem/Subsystem1/Torque Distribution/MPC/Polytopic Constraints ==
  In Bus Element5 : Inport  PortName=hv
  In Bus Element7 : Inport  PortName=hv
  In Bus Element35 : Inport  Port=2  PortName=brake_signal
  In Bus Element4 : Inport  Port=2  PortName=brake_signal
  In Bus Element{1..3,6} (4 alike) : Inport  Port=3  PortName=driver_inputs
  In Bus torque_map : Inport  Port=4  PortName=Car_Settings
  In Bus Element : Inport  Port=5  PortName=mz  Element=ub
  In Bus Element8 : Inport  Port=5  PortName=mz  Element=lb
  Bus Element In1 : Inport  Port=6  PortName=InBus
  Driver Inputs : Subsystem
      settings: PortSchema="{\"entries\":[{\"content\":{\"sides\":[{\"content\":{\"connectorIds\":[\"In1\",\"In2\",\"In3\",\"In4\"]},\"type\":\"ConnectorPlacement.EquallySpacedRectSide\",\"uuid\":\"334783ee-11f3-4144-8a14-28dc56086a4b\"},{\"content\":{\"connectorIds\":[\"Out1\"],\"side\":\"RIGHT\"},\"type\":\"ConnectorPlacement.EquallySpacedRectSide\",\"uuid\":\"49c8e620-bd09-4fee-a8d6-6c7a5f6563c1\"},{\"content\":{\"connectorIds\":[\"Out2\"],\"side\":\"TOP\"},\"type\":\"ConnectorPlacement.EquallySpacedRectSide\",\"uuid\":\"cef52ef8-f6f7-4321-a9c9-502de0ffc851\"}]},\"type\":\"ConnectorPlacement.EquallySpacedConnector\",\"uuid\":\"45428ca6-b9a3-4f64-8f7b-2072997d615d\"}],\"packageUris\":[\"http://schema.mathworks.com/mf0/Connector/R2020b\"],\"version\":\"1.0\"}"
  Driver g : Subsystem
      settings: PortSchema="{\"entries\":[{\"content\":{\"sides\":[{\"content\":{\"connectorIds\":[\"In1\",\"In2\",\"In3\"]},\"type\":\"ConnectorPlacement.EquallySpacedRectSide\",\"uuid\":\"52593113-81e3-4b2d-919c-0421b1274de7\"},{\"content\":{\"connectorIds\":[\"Out1\",\"Out2\"],\"side\":\"RIGHT\"},\"type\":\"ConnectorPlacement.EquallySpacedRectSide\",\"uuid\":\"003691be-7065-493d-8a97-6bcaaf8c0f8d\"},{\"content\":{\"connectorIds\":[\"Out3\"],\"side\":\"TOP\"},\"type\":\"ConnectorPlacement.EquallySpacedRectSide\",\"uuid\":\"77e10d31-2af4-42f4-ba5d-4e60bb02d914\"}]},\"type\":\"ConnectorPlacement.EquallySpacedConnector\",\"uuid\":\"ad322a89-c7fc-4aff-bfd3-29198c6c5477\"}],\"packageUris\":[\"http://schema.mathworks.com/mf0/Connector/R2020b\"],\"version\":\"1.0\"}"
  Mux : Mux  Inputs=5
  Mux1 : Mux  Inputs=5
  Power Limits Negative : Subsystem
  Power Limits Positive : Subsystem
  Subsystem : Subsystem
  Subsystem1 : Subsystem
  lg : Outport
  ug : Outport  Port=2
  Out Bus Element1 : Outport  Port=3  PortName=TV_Info  Element=Driver_Inputs
  Out Bus Element2 : Outport  Port=3  PortName=TV_Info  Element=ug
  Out Bus Element3 : Outport  Port=3  PortName=TV_Info  Element=lg
  Out Bus Element4 : Outport  Port=3  PortName=TV_Info  Element=Driver_g
  wires:
  In Bus Element3/1 -> Subsystem1/1(driver_inputs)
  In Bus Element1/1 -> Subsystem/1(driver_inputs)
  Power Limits Negative/1(lg_power) -> Mux1/2
  Subsystem1/1(Out1) -> Mux1/4, Mux1/3
  Subsystem/1(Out1) -> Mux/4, Mux/3
  Mux/1 -> Out Bus Element2/1, ug/1
  Mux1/1 -> lg/1, Out Bus Element3/1
  In Bus Element35/1 -> Driver Inputs/1(brake_signal)
  In Bus Element2/1 -> Driver Inputs/2(driver_inputs)
  In Bus torque_map/1 -> Driver Inputs/3(Car_Settings)
  Driver Inputs/1(percentage) -> Driver g/2(percentage)
  In Bus Element4/1 -> Driver g/1(brake_signal)
  In Bus Element6/1 -> Driver g/3(driver_inputs)
  In Bus Element5/1 -> Power Limits Positive/1(hv)  "hv"
  Power Limits Positive/1(ug_power) -> Mux/2
  In Bus Element7/1 -> Power Limits Negative/1(hv)  "hv"
  Driver Inputs/2(TV_Info) -> Out Bus Element1/1
  Driver g/3(TV_Info) -> Out Bus Element4/1
  In Bus Element/1 -> Mux/5
  In Bus Element8/1 -> Mux1/5
  Driver g/1(ug_driver) -> Mux/1
  Driver g/2(lg_driver) -> Mux1/1
  Bus Element In1/1 -> Driver Inputs/4(InBus)

== system TVModel/Subsystem/Subsystem1/Torque Distribution/MPC/Polytropic Matrix ==
  In Bus Element1 : Inport  PortName=dynamics_data
  Torque : Inport  Port=2
  In Bus Element8 : Inport  Port=3  PortName=front_wheel_angles  Element=different_axis
  Efficiency limit : Subsystem
  MATLAB Function : MATLAB Function  TreatAsAtomicUnit=on
  c : Outport
  Out Bus Element22 : Outport  Port=2  PortName=TV_Info  Element=c
  wires:
  In Bus Element8/1 -> MATLAB Function/2(delta)
  MATLAB Function/1(y) -> Out Bus Element22/1, c/1
  Efficiency limit/1(efficiency_limit) -> MATLAB Function/1(Limit)
  In Bus Element1/1 -> Efficiency limit/2(dynamics_data)
  Torque/1 -> Efficiency limit/1(motor_torque)

== system TVModel/Subsystem/Subsystem1/Torque Distribution/MPC/Power Calculation Pre ==
  Motor_Torque : Inport  OutDataTypeStr=double  PortDimensions=4
  In Bus Element34 : Inport  Port=2  PortName=dynamics_data  Element=omega_wheels
  In Bus Element2 : Inport  Port=2  PortName=dynamics_data  Element=omega_wheels
  "     " : Gain  Gain=TV.LV.inv_efficiency
  "      " : Gain  Gain=1/TV.LV.inv_efficiency
  Divide : Product  Inputs=*/*
  Gain2 : Gain  Gain=TV.CAR.Tau
  Power to engines : Subsystem
  Saturation : Saturate  UpperLimit=19900*pi/30  LowerLimit=100*pi/30
  Sum of Elements : Sum  Inputs=+
  Switch3 : Switch  Criteria=u2 > Threshold  SaturateOnIntegerOverflow=off  InputSameDT=off
  Terminator : Terminator
  wires:
  Power to engines/1(Efficiency) -> "      "/1, "     "/1
  "      "/1 -> Switch3/3  "Braking"
  "     "/1 -> Switch3/1  "Driving"
  Motor_Torque/1 -> Divide/3, Power to engines/2(Torque)
  In Bus Element34/1 -> Gain2/1
  Gain2/1 -> Saturation/1
  In Bus Element2/1 -> Switch3/2
  Sum of Elements/1 -> Terminator/1  "p_el_pre"
  Saturation/1 -> Divide/1, Power to engines/1(omega_motor)
  Switch3/1 -> Divide/2
  Divide/1 -> Sum of Elements/1

== system TVModel/Subsystem/Subsystem1/Torque Distribution/MPC/Slack variables Weights  ==
  Constant : Constant  Value=[1e3;1e-3;1e-3]
  zl_e : Outport
  zu_e : Outport  Port=2
  wires:
  Constant/1 -> zl_e/1, zu_e/1

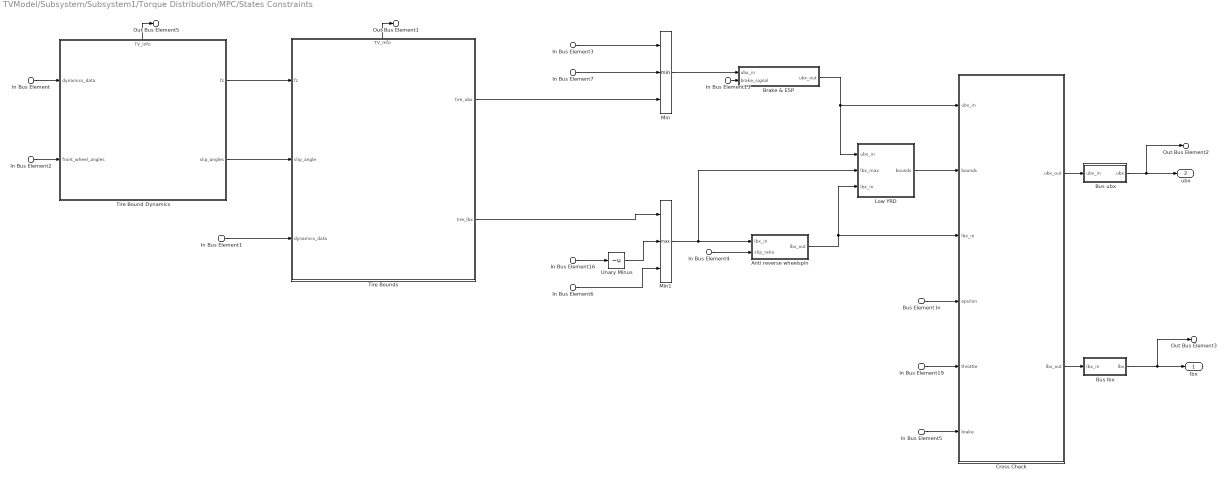
== system TVModel/Subsystem/Subsystem1/Torque Distribution/MPC/States Constraints ==
  In Bus Element2 : Inport  PortName=front_wheel_angles
  In Bus Element16 : Inport  Port=2  PortName=torque_limits  Element=t_limit_negative
  In Bus Element3 : Inport  Port=2  PortName=torque_limits  Element=t_limit_positive
  In Bus Element6 : Inport  Port=3  PortName=TC_Torque  Element=Regen
  In Bus Element7 : Inport  Port=3  PortName=TC_Torque  Element=Traction
  In Bus Element : Inport  Port=4  PortName=dynamics_data
  In Bus Element1 : Inport  Port=4  PortName=dynamics_data
  In Bus Element4 : Inport  Port=5  PortName=slip_ratio
  In Bus Element13 : Inport  Port=6  PortName=brake_signal
  Bus Element In : Inport  Port=7  PortName=epsilon
  In Bus Element5 : Inport  Port=8  PortName=driver_inputs  Element=brake
  In Bus Element19 : Inport  Port=8  PortName=driver_inputs  Element=throttle
  Anti reverse wheelspin : Subsystem
  Brake & ESP : Subsystem
  Bus lbx : Subsystem
  Bus ubx : Subsystem
  Cross Check : MATLAB Function  TreatAsAtomicUnit=on
  Low YRD : Subsystem
  Min : MinMax  Inputs=3
  Min1 : MinMax  Function=max  Inputs=3
  Tire Bound Dynamics : Subsystem
      settings: PortSchema="{\"entries\":[{\"content\":{\"sides\":[{\"content\":{\"connectorIds\":[\"In1\",\"In2\"]},\"type\":\"ConnectorPlacement.EquallySpacedRectSide\",\"uuid\":\"c905e0d5-9d26-4c00-bd7e-07ee0633c160\"},{\"content\":{\"connectorIds\":[\"Out1\",\"Out2\"],\"side\":\"RIGHT\"},\"type\":\"ConnectorPlacement.EquallySpacedRectSide\",\"uuid\":\"37cd4095-0f8c-481f-b8de-23350fc0b3e2\"},{\"content\":{\"connectorIds\":[\"Out3\"],\"side\":\"TOP\"},\"type\":\"ConnectorPlacement.EquallySpacedRectSide\",\"uuid\":\"585cff9f-4d8e-4579-999e-dff949f4791c\"}]},\"type\":\"ConnectorPlacement.EquallySpacedConnector\",\"uuid\":\"48494429-6ae2-4bc0-abe5-17d5f904d891\"}],\"packageUris\":[\"http://schema.mathworks.com/mf0/Connector/R2020b\"],\"version\":\"1.0\"}"
  Tire Bounds : Subsystem
      settings: PortSchema="{\"entries\":[{\"content\":{\"sides\":[{\"content\":{\"connectorIds\":[\"In1\",\"In2\",\"In3\"]},\"type\":\"ConnectorPlacement.EquallySpacedRectSide\",\"uuid\":\"c905e0d5-9d26-4c00-bd7e-07ee0633c160\"},{\"content\":{\"connectorIds\":[\"Out1\",\"Out2\"],\"side\":\"RIGHT\"},\"type\":\"ConnectorPlacement.EquallySpacedRectSide\",\"uuid\":\"37cd4095-0f8c-481f-b8de-23350fc0b3e2\"},{\"content\":{\"connectorIds\":[\"Out3\"],\"side\":\"TOP\"},\"type\":\"ConnectorPlacement.EquallySpacedRectSide\",\"uuid\":\"585cff9f-4d8e-4579-999e-dff949f4791c\"}]},\"type\":\"ConnectorPlacement.EquallySpacedConnector\",\"uuid\":\"48494429-6ae2-4bc0-abe5-17d5f904d891\"}],\"packageUris\":[\"http://schema.mathworks.com/mf0/Connector/R2020b\"],\"version\":\"1.0\"}"
  Unary Minus : UnaryMinus
  lbx : Outport
  ubx : Outport  Port=2
  Out Bus Element2 : Outport  Port=3  PortName=TV_Info  Element=ubx
  Out Bus Element3 : Outport  Port=3  PortName=TV_Info  Element=lbx
  Out Bus Element5 : Outport  Port=3  PortName=TV_Info  Element=Tire_Bound_Dynamics
  Out Bus Element1 : Outport  Port=3  PortName=TV_Info  Element=Tire_Bounds
  wires:
  In Bus Element19/1 -> Cross Check/5(throttle)
  Bus Element In/1 -> Cross Check/4(epsilon)
  In Bus Element7/1 -> Min/2
  Min1/1 -> Anti reverse wheelspin/1(lbx_in), Low YRD/2(lbx_max)
  Low YRD/1(bounds) -> Cross Check/2(bounds)
  Anti reverse wheelspin/1(lbx_out) -> Cross Check/3(lbx_in), Low YRD/3(lbx_in)
  Bus lbx/1(lbx) -> lbx/1, Out Bus Element3/1
  Bus ubx/1(ubx) -> Out Bus Element2/1, ubx/1
  In Bus Element3/1 -> Min/1
  In Bus Element16/1 -> Unary Minus/1
  Cross Check/1(ubx_out) -> Bus ubx/1(ubx_in)
  Cross Check/2(lbx_out) -> Bus lbx/1(lbx_in)
  Unary Minus/1 -> Min1/2
  In Bus Element/1 -> Tire Bound Dynamics/1(dynamics_data)
  In Bus Element2/1 -> Tire Bound Dynamics/2(front_wheel_angles)
  Tire Bound Dynamics/3(TV_Info) -> Out Bus Element5/1
  Tire Bound Dynamics/2(slip_angles) -> Tire Bounds/2(slip_angle)
  Tire Bound Dynamics/1(fz) -> Tire Bounds/1(fz)
  Tire Bounds/3(TV_Info) -> Out Bus Element1/1
  In Bus Element1/1 -> Tire Bounds/3(dynamics_data)
  Tire Bounds/1(tire_ubx) -> Min/3
  Tire Bounds/2(tire_lbx) -> Min1/1
  Min/1 -> Brake & ESP/1(ubx_in)
  Brake & ESP/1(ubx_out) -> Cross Check/1(ubx_in), Low YRD/1(ubx_in)
  In Bus Element13/1 -> Brake & ESP/2(brake_signal)
  In Bus Element4/1 -> Anti reverse wheelspin/2(slip_ratio)
  In Bus Element5/1 -> Cross Check/6(brake)
  In Bus Element6/1 -> Min1/3

== system TVModel/Subsystem/Subsystem1/Torque Distribution/MPC/USEFUL STUFFFF ==
  In Bus Element10 : Inport  PortName=front_wheels_steering  Element=single_axis
  Abs : Abs  Commented=on  SaturateOnIntegerOverflow=off
  Chart : Stateflow chart  Commented=on  TreatAsAtomicUnit=on
  Constant3 : Constant  Commented=on  Value=TV.SIGNALS.SETTINGS.steer_threshold
  Constant5 : Constant  Commented=on  Value=TV.SIGNALS.SETTINGS.steer_relay_amplitude
  Extended Kalman Filter : Subsystem  Commented=on
  Non-Linear Activation : MATLAB Function  Commented=on  TreatAsAtomicUnit=on
  Power Limiter : Subsystem  Commented=on
  Power flag : Subsystem  Commented=on
  Radians to Degrees : simulink_extras/Transformations/Radians to Degrees  Commented=on
  States Selector : Subsystem  Commented=on
  Subsystem : Subsystem  Commented=on
  Subsystem1 : Subsystem  Commented=on
  Yrd 0 When Steering 0 : Subsystem  Commented=on
      mask Display: image('Mask_Icon\On_Off.png'); % Use "Edit Image" on toolstrip to change.
  lbu_dot : Subsystem  Commented=on
  wires:
  Power flag/1(Output) -> ?
  Subsystem/1(Output) -> ?
  Abs/1 -> Chart/1(front_wheels_steering)
  In Bus Element10/1 -> Radians to Degrees/1
  Constant5/1 -> Chart/2(semi_amplitude)
  Radians to Degrees/1 -> Abs/1
  Constant3/1 -> Chart/3(steer_threshold)

== system TVModel/Subsystem/Subsystem1/Torque Distribution/MPC/Useful Calculations ==
  In Bus Element16 : Inport  PortName=dynamics_data
  In Bus Element18 : Inport  Port=2  PortName=front_wheel_angles  Element=different_axis
  Inport : Inport  Port=3
  Inport1 : InportShadow  Port=3
  MATLAB Function : MATLAB Function  TreatAsAtomicUnit=on
  Power Calculation Post : Subsystem
  Terminator : Terminator
  wires:
  Inport1/1 -> MATLAB Function/1(T)
  Inport/1 -> Power Calculation Post/2(Motor_Torque)
  In Bus Element18/1 -> MATLAB Function/2(delta)
  MATLAB Function/1(y) -> Terminator/1  "Mz_Real"
  In Bus Element16/1 -> Power Calculation Post/1(dynamics_data)

== system TVModel/Subsystem/Subsystem1/Torque Distribution/MPC/Weights Generation ==
  In Bus Element1 : Inport  PortName=dynamics_data
  Torque : Inport  Port=2
  Constant : Constant  Value=TV.SIGNALS.SETTINGS.DerivativeTorqueWeight*ones(4,1)
  Constant1 : Constant  VectorParams1D=off
  Constant2 : Constant  Value=TV.SIGNALS.SETTINGS.TorqueWeight*ones(4,1)
  Demux : Demux
  Demux1 : Demux
  Efficiency limit : Subsystem
  MATLAB Function : MATLAB Function  TreatAsAtomicUnit=on
  Mux : Mux  Inputs=TV.MPC.ny
  Terminator : Terminator
  r1 : Constant  Value=TV.SIGNALS.SETTINGS.wYawWeight
  vx : Constant  Value=0
  vy : Constant  Value=TV.SIGNALS.SETTINGS.VyWeight
  w : Outport
  Out Bus Element3 : Outport  Port=2  PortName=TV_Info  Element=w
  wires:
  Constant/1 -> Demux1/1
  Demux1/2 -> Mux/9
  Demux1/4 -> Mux/11
  Demux1/1 -> Mux/8
  Demux1/3 -> Mux/10
  Mux/1 -> MATLAB Function/1(u)
  vy/1 -> Mux/2
  vx/1 -> Mux/1
  MATLAB Function/1(y) -> Out Bus Element3/1, w/1
  Demux/1 -> Mux/4
  Demux/2 -> Mux/5
  Demux/4 -> Mux/7
  Demux/3 -> Mux/6
  Torque/1 -> Efficiency limit/1(motor_torque)
  In Bus Element1/1 -> Efficiency limit/2(dynamics_data)
  r1/1 -> Mux/3
  Constant1/1 -> MATLAB Function/2(deltaAxle)
  Constant2/1 -> Demux/1
  Efficiency limit/1(efficiency_limit) -> Terminator/1

== system TVModel/Subsystem/Subsystem1/Torque Distribution/Reference Tracking/YRD_LUT_-1 ==
  front_wheel_angle : Inport
  vx : Inport  Port=2
  Action Port : ActionPort  ActionPortLabel=elseif(u1 ==4)
  Abs : Abs  SaturateOnIntegerOverflow=off
  Cast3 : DataTypeConversion  Commented=on  OutDataTypeStr=single  SaturateOnIntegerOverflow=off  RndMeth=Floor
  Divide : Product  Inputs=*/
  Divide1 : Product  Inputs=*/
  Divide2 : Product  Inputs=**
  LUT_-3 : Lookup_n-D  BreakpointsForDimension1=TV.LUT.Yrd_LUT.LUT_vectors.delta_vector  BreakpointsForDimension2=TV.LUT.Yrd_LUT.LUT_vectors.v_vector  Table=single(TV.LUT.Yrd_LUT.LUT_neg3.ay_matrix)  InternalRulePriority=Speed  RndMeth=Simplest
      settings: InputPortMap=u0,u1
  Saturation : Saturate  UpperLimit=inf  LowerLimit=3
  yrd : Outport
  wires:
  Divide1/1 -> Divide2/1  "normalized_front_wheel_angle"
  Divide2/1 -> yrd/1  "yrd"
  Saturation/1 -> LUT_-3/2, Divide/2  "vx"
  vx/1 -> Saturation/1
  LUT_-3/1 -> Divide/1  "a"
  Divide/1 -> Divide2/2
  Abs/1 -> LUT_-3/1, Divide1/2  "absolute_front_wheel_angle"
  front_wheel_angle/1 -> Abs/1, Divide1/1

== system TVModel/Subsystem/Subsystem1/Torque Distribution/Reference Tracking/YRD_LUT_-1.1 ==
  front_wheel_angle : Inport
  vx : Inport  Port=2
  Action Port : ActionPort  ActionPortLabel=elseif(u1 ==3)
  Abs : Abs  SaturateOnIntegerOverflow=off
  Cast3 : DataTypeConversion  Commented=on  OutDataTypeStr=single  SaturateOnIntegerOverflow=off  RndMeth=Floor
  Divide : Product  Inputs=*/
  Divide1 : Product  Inputs=*/
  Divide2 : Product  Inputs=**
  LUT_-1.5 : Lookup_n-D  BreakpointsForDimension1=TV.LUT.Yrd_LUT.LUT_vectors.delta_vector  BreakpointsForDimension2=TV.LUT.Yrd_LUT.LUT_vectors.v_vector  Table=single(TV.LUT.Yrd_LUT.LUT_neg1_5.ay_matrix)  InternalRulePriority=Speed  RndMeth=Simplest
      settings: InputPortMap=u0,u1
  Saturation : Saturate  UpperLimit=inf  LowerLimit=3
  yrd : Outport
  wires:
  Divide/1 -> Divide2/2
  LUT_-1.5/1 -> Divide/1
  Saturation/1 -> LUT_-1.5/2, Divide/2  "vx"
  Abs/1 -> LUT_-1.5/1, Divide1/2  "absolute_front_wheel_angle"
  Divide2/1 -> yrd/1  "yrd"
  Divide1/1 -> Divide2/1  "normalized_front_wheel_angle"
  vx/1 -> Saturation/1
  front_wheel_angle/1 -> Abs/1, Divide1/1

== system TVModel/Subsystem/Subsystem1/Torque Distribution/Reference Tracking/YRD_LUT_-1.5 ==
  front_wheel_angle : Inport
  vx : Inport  Port=2
  Action Port : ActionPort  ActionPortLabel=elseif(u1 ==3)
  Abs : Abs  SaturateOnIntegerOverflow=off
  Cast3 : DataTypeConversion  Commented=on  OutDataTypeStr=single  SaturateOnIntegerOverflow=off  RndMeth=Floor
  Divide : Product  Inputs=*/
  Divide1 : Product  Inputs=*/
  Divide2 : Product  Inputs=**
  LUT_-1.5 : Lookup_n-D  BreakpointsForDimension1=TV.LUT.Yrd_LUT.LUT_vectors.delta_vector  BreakpointsForDimension2=TV.LUT.Yrd_LUT.LUT_vectors.v_vector  Table=single(TV.LUT.Yrd_LUT.LUT_neg1_5.ay_matrix)  InternalRulePriority=Speed  RndMeth=Simplest
      settings: InputPortMap=u0,u1
  Saturation : Saturate  UpperLimit=inf  LowerLimit=3
  yrd : Outport
  wires:
  front_wheel_angle/1 -> Divide1/1, Abs/1
  vx/1 -> Saturation/1
  Divide1/1 -> Divide2/1  "normalized_front_wheel_angle"
  Divide2/1 -> yrd/1  "yrd"
  Abs/1 -> Divide1/2, LUT_-1.5/1  "absolute_front_wheel_angle"
  Saturation/1 -> Divide/2, LUT_-1.5/2  "vx"
  LUT_-1.5/1 -> Divide/1
  Divide/1 -> Divide2/2
